simulink model "depth_lin"  (R2023b)
settings: Solver=VariableStepAuto  StartTime=0.0  StopTime=100  RelTol=1e-3
settings Model: Creator=fabio  LastModifiedBy=fabio

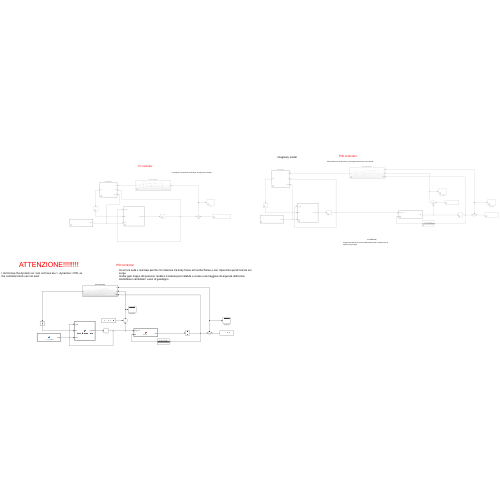
[thumbnail: Simulink's stored preview of the top-level diagram]
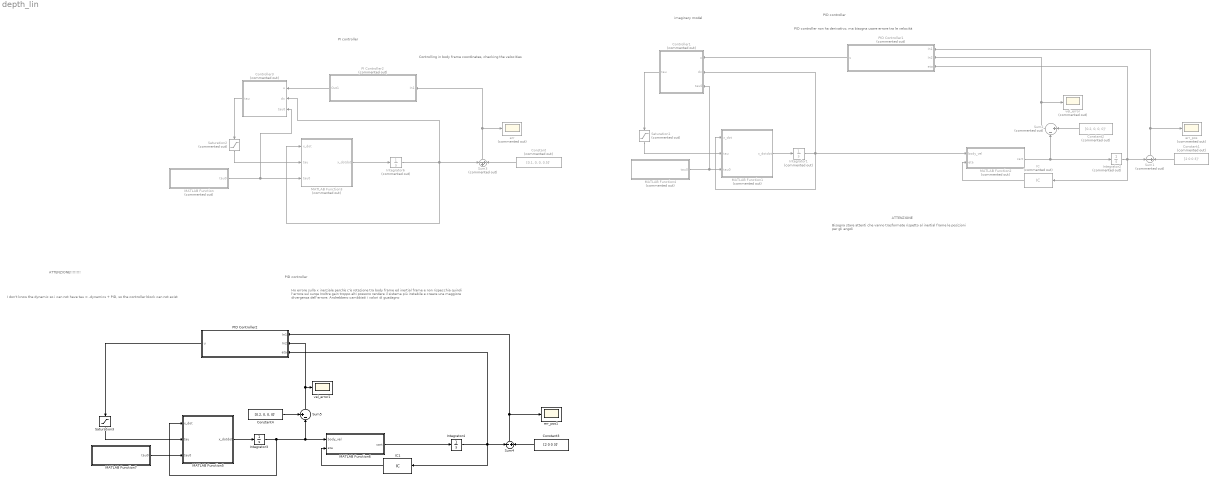
== system depth_lin ==
  note: Ho errore sulla x inerziale perchè c'è rotazione tra body frame ed inertial frame e non rispecchia quindi l'errore sul surge
      | Inoltre gain troppo alti possono rendere il sistema più instabile e creare una maggiore divergenza dell'errore.
      | Andrebbero cambbiati i valori di guadagno
  note: imaginary model
  note: I don't know the dynamic so i can not have tau = -dynamics + PID, so the controller block can not exist
  note: ATTENZIONE!!!!!!!!
  note: PID controller non ha derivativo, ma bisogna usare errore tra le velocità
  note: Controlling in body frame coordinates, checking the velocities
  note: PID controller
  note: PI controller
  note: Bisogna stare attenti che vanno trasformate rispetto al inertial frame le posizioni per gli angoli
  note: ATTENZIONE
  note: PID controller
  Constant : Constant  Commented=on  Value=[0.1, 0, 0, 0.5]'
  Constant1 : Constant  Commented=on  Value=[2 0 0 3]'
  Constant2 : Constant  Commented=on  Value=[0.2, 0, 0, 0]'
  Constant3 : Constant  Value=[2 0 0 3]'
  Constant4 : Constant  Value=[0.2, 0, 0, 0]'
  Controller1 : MATLAB Function  Commented=on  TreatAsAtomicUnit=on
  Controller3 : MATLAB Function  Commented=on  TreatAsAtomicUnit=on
  IC : InitialCondition  Commented=on  Value=[1, 0, 1, 0.5]'
  IC1 : InitialCondition  Value=[1, 0, 0, 0.5]'
  Integrator1 : Integrator  Commented=on
  Integrator2 : Integrator  Commented=on
  Integrator3 : Integrator
  Integrator4 : Integrator
  Integrator6 : Integrator  Commented=on
  MATLAB Function : MATLAB Function  Commented=on  TreatAsAtomicUnit=on
  MATLAB Function1 : MATLAB Function  Commented=on  TreatAsAtomicUnit=on
  MATLAB Function2 : MATLAB Function  Commented=on  TreatAsAtomicUnit=on
  MATLAB Function3 : MATLAB Function  Commented=on  TreatAsAtomicUnit=on
  MATLAB Function4 : MATLAB Function  Commented=on  TreatAsAtomicUnit=on
  MATLAB Function5 : MATLAB Function  TreatAsAtomicUnit=on
  MATLAB Function6 : MATLAB Function  TreatAsAtomicUnit=on
  MATLAB Function7 : MATLAB Function  TreatAsAtomicUnit=on
  PI Controller2 : Subsystem  Commented=on
  PID Controller1 : Subsystem  Commented=on
  PID Controller2 : Subsystem
  Saturation1 : Saturate  Commented=on  UpperLimit=20000  LowerLimit=-20000
  Saturation2 : Saturate  Commented=on  UpperLimit=20000  LowerLimit=-20000
  Saturation3 : Saturate  UpperLimit=20000  LowerLimit=-20000
  Sum1 : Sum  Commented=on  Inputs=-+
  Sum2 : Sum  Commented=on  Inputs=||+|-
  Sum3 : Sum  Commented=on  Inputs=-++
  Sum4 : Sum  Inputs=-+
  Sum5 : Sum  Inputs=+-|
  err : Scope  Commented=on
  err_pos : Scope  Commented=on
  err_pos1 : Scope
  vel_error : Scope  Commented=on
  vel_error1 : Scope
  wires:
  Controller3/1(tau) -> Saturation2/1
  Sum3/1 -> err/1, PI Controller2/1(In1)
  Saturation2/1 -> MATLAB Function3/2(tau)
  PI Controller2/1(Out1) -> Controller3/1(u)
  MATLAB Function3/1(x_dotdot) -> Integrator6/1
  Integrator6/1 -> Controller3/2(dx), MATLAB Function3/1(x_dot), Sum3/1
  MATLAB Function2/1(cart) -> Sum2/2, Integrator2/1
  Controller1/1(tau) -> Saturation1/1
  Integrator2/1 -> PID Controller1/3(eta), IC/1, Sum1/1
  Saturation1/1 -> MATLAB Function1/2(tau)
  Integrator1/1 -> MATLAB Function2/1(body_vel), MATLAB Function1/1(x_dot), Controller1/2(dx)
  MATLAB Function1/1(x_dotdot) -> Integrator1/1
  Sum1/1 -> PID Controller1/1(In1), err_pos/1
  MATLAB Function/1(tau0) -> MATLAB Function3/3(tau0), Controller3/3(tau0)
  Constant/1 -> Sum3/3
  MATLAB Function4/1(tau0) -> MATLAB Function1/3(tau0), Controller1/3(tau0)
  Constant1/1 -> Sum1/2
  Sum2/1 -> PID Controller1/2(In2), vel_error/1
  Constant2/1 -> Sum2/1
  PID Controller1/1(u) -> Controller1/1(u)
  IC/1 -> MATLAB Function2/2(eta)
  Constant4/1 -> Sum5/1
  Constant3/1 -> Sum4/2
  Saturation3/1 -> MATLAB Function5/2(tau)
  Integrator3/1 -> MATLAB Function6/1(body_vel), Sum5/2, MATLAB Function5/1(x_dot)
  Sum5/1 -> PID Controller2/2(In2), vel_error1/1
  MATLAB Function5/1(x_dotdot) -> Integrator3/1
  IC1/1 -> MATLAB Function6/2(eta)
  MATLAB Function7/1(tau0) -> MATLAB Function5/3(tau0)
  Integrator4/1 -> PID Controller2/3(eta), IC1/1, Sum4/1
  Sum4/1 -> PID Controller2/1(In1), err_pos1/1
  MATLAB Function6/1(cart) -> Integrator4/1
  PID Controller2/1(u) -> Saturation3/1

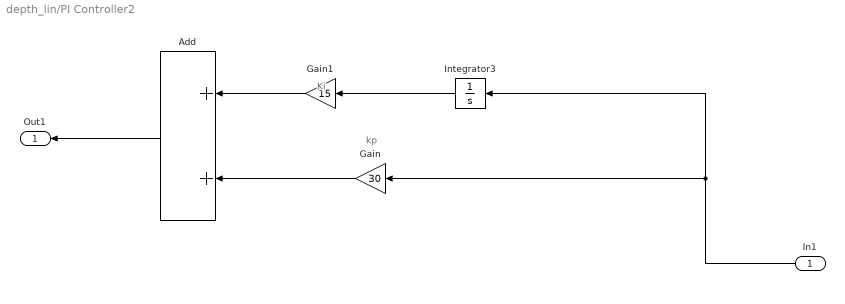
== system depth_lin/PI Controller2 ==
  note: Ki
  note: kp
  In1 : Inport
  Add : Sum
  Gain : Gain  Gain=30
  Gain1 : Gain  Gain=15
  Integrator3 : Integrator
  Out1 : Outport
  wires:
  Gain/1 -> Add/2
  Integrator3/1 -> Gain1/1
  In1/1 -> Integrator3/1, Gain/1
  Add/1 -> Out1/1
  Gain1/1 -> Add/1

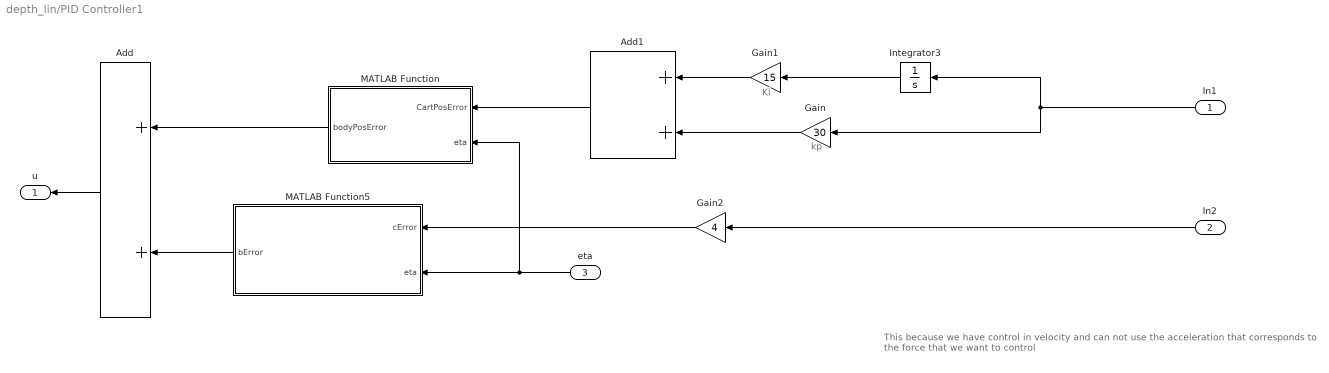
== system depth_lin/PID Controller1 ==
  note: This because we have control in velocity and can not use the acceleration that corresponds to the force that we want to control
  note: Ki
  note: kp
  In1 : Inport
  In2 : Inport  Port=2
  eta : Inport  Port=3
  Add : Sum
  Add1 : Sum
  Gain : Gain  Gain=30
  Gain1 : Gain  Gain=15
  Gain2 : Gain  Gain=4
  Integrator3 : Integrator
  MATLAB Function : MATLAB Function  TreatAsAtomicUnit=on
  MATLAB Function5 : MATLAB Function  TreatAsAtomicUnit=on
  u : Outport
  wires:
  Integrator3/1 -> Gain1/1
  In1/1 -> Integrator3/1, Gain/1
  Add/1 -> u/1
  In2/1 -> Gain2/1
  Gain1/1 -> Add1/1
  Gain/1 -> Add1/2
  Gain2/1 -> MATLAB Function5/1(cError)
  MATLAB Function5/1(bError) -> Add/2
  eta/1 -> MATLAB Function/2(eta), MATLAB Function5/2(eta)
  Add1/1 -> MATLAB Function/1(CartPosError)
  MATLAB Function/1(bodyPosError) -> Add/1

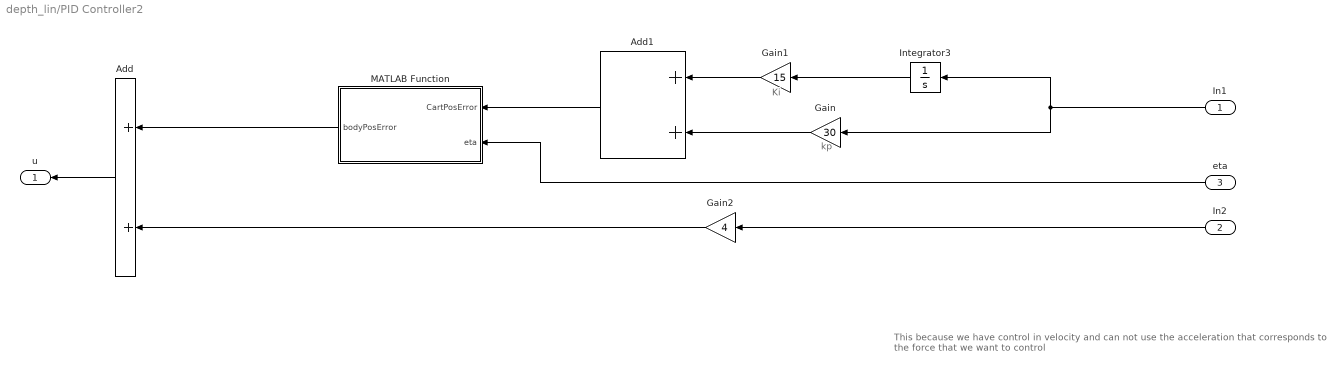
== system depth_lin/PID Controller2 ==
  note: This because we have control in velocity and can not use the acceleration that corresponds to the force that we want to control
  note: Ki
  note: kp
  In1 : Inport
  In2 : Inport  Port=2
  eta : Inport  Port=3
  Add : Sum
  Add1 : Sum
  Gain : Gain  Gain=30
  Gain1 : Gain  Gain=15
  Gain2 : Gain  Gain=4
  Integrator3 : Integrator
  MATLAB Function : MATLAB Function  TreatAsAtomicUnit=on
  u : Outport
  wires:
  Integrator3/1 -> Gain1/1
  In1/1 -> Integrator3/1, Gain/1
  Add/1 -> u/1
  In2/1 -> Gain2/1
  Gain1/1 -> Add1/1
  Gain/1 -> Add1/2
  Gain2/1 -> Add/2
  eta/1 -> MATLAB Function/2(eta)
  Add1/1 -> MATLAB Function/1(CartPosError)
  MATLAB Function/1(bodyPosError) -> Add/1

== matlab function depth_lin/MATLAB Function7 ==
  data: tau0 output
function tau0 = tau0Computation()
    % updated to medusa model
    m = 30;
    I = 4.14;
    g = 9.81;
    WB = -0.8339; % Buoyancy
    
    % x initial
    speed0 = [0.1, 0, 0, 0]';

    % Added mass
    tau_a = [-25; -2.325; -8.690; -19.4311]; % kl_dot

    % Restoring forces
    tau_r = [-0.2; -55.117; -4.14; 33.6804]; % kl

    % Hydrodynamic forces
    tau_d = [-19.5; -147.9; -6.23; -89.4105]; % kl_modl

    % Virtual mass
    mv = [m; m; I; m] - tau_a;

    % Dissatipative forces
    dv = -tau_r - 2*tau_d .* abs(speed0);
    
    % tau0 computation
    tau0 = zeros(4,1);
    tau0(1) = dv(1)*speed0(1) - mv(2)*speed0(2)*speed0(3);
    tau0(2) = 0; % can do also the equations
    tau0(3) = dv(3)*speed0(3) - (mv(1) - mv(2))*speed0(1)*speed0(2);
    tau0(4) = -dv(4)*speed0(4) - WB;
end

== matlab function depth_lin/PID Controller2/MATLAB Function ==
  data: CartPosError input; bodyPosError output; eta input
function bodyPosError = Rotation(CartPosError, eta)
    angle = eta(3);
    bodyPosError = zeros(4,1);
    rot = [cos(angle), -sin(angle)
            sin(angle), cos(angle)];

    bodyPosError(1:2) = rot' * CartPosError(1:2);
    bodyPosError(3:4) = CartPosError(3:4);
end

== matlab function depth_lin/Controller1 ==
  data: u input; dx input; tau output; tau0 input
function tau = controller(u, dx, tau0)
    % updated to medusa model
    m = 30;
    I = 4.14;
    K = 1;
    
    % x initial
    speed0 = [0.1, 0, 0, 0]';

    % Added mass
    tau_a = [-25; -2.325; -8.690; -19.4311]; % kl_dot

    % Restoring forces
    tau_r = [-0.2; -55.117; -4.14; 33.6804]; % kl

    % Hydrodynamic forces
    tau_d = [-19.5; -147.9; -6.23; -89.4105]; % kl_modl

    % Virtual mass
    mv = [m; m; I; m] - tau_a;

    % Dissatipative forces
    dv = -tau_r - 2*tau_d .*abs(speed0);
    
    % delta velocities
    delta = dx - speed0;
    % Accelerations
    % 3 DOF MODEL
    tau = zeros(4,1);
    % Tested tau. Which is the best methods??
    % tau(1) = mv(1)*K*u(1) + dv(1)*dx(1) - mv(2)*speed0(2)*dx(3) - mv(2)*speed0(3)*dx(2);
    % tau(2) = 0; % can do also the equations
    % tau(3) = mv(3)*K*u(3) + dv(3)*dx(3) - (mv(1) - mv(2))*speed0(1)*dx(2) - (mv(1) - mv(2))*speed0(2)*dx(1);
    % % Considering also depth (heavy)
    % tau(4) =  mv(4)*K*u(4) - dv(4)*dx(4);

    % Consider also deltas and initial tau
    tau(1) = mv(1)*K*u(1) + dv(1)*delta(1) - mv(2)*speed0(2)*delta(3) - mv(2)*speed0(3)*delta(2) + tau0(1);
    tau(2) = 0; % can do also the equations
    tau(3) = mv(3)*K*u(3) + dv(3)*delta(3) - (mv(1) - mv(2))*speed0(1)*delta(2) - (mv(1) - mv(2))*speed0(2)*delta(1) + tau0(3);
    % Considering also depth (heavy)
    tau(4) =  mv(4)*K*u(4) - dv(4)*delta(4) + tau0(4);
end

== matlab function depth_lin/MATLAB Function1 ==
  data: x_dot input; tau input; tau0 input; x_dotdot output
function x_dotdot = vehicle_dynamics_matrix(x_dot, tau, tau0)
    % updated to medusa model
    m = 30;
    I = 4.14;
    
    % x initial
    speed0 = [0.1, 0, 0, 0]';

    % Added mass
    tau_a = [-25; -2.325; -8.690; -19.4311]; % kl_dot

    % Restoring forces
    tau_r = [-0.2; -55.117; -4.14; 33.6804]; % kl

    % Hydrodynamic forces
    tau_d = [-19.5; -147.9; -6.23; -89.4105]; % kl_modl

    % Virtual mass
    mv = [m; m; I; m] - tau_a;

    % Dissatipative forces
    dv = -tau_r - 2*tau_d .* abs(speed0);

    delta = x_dot - speed0;

    % Accelerations
    % 3 DOF MODEL Linearized
    x_dotdot = zeros(4,1);
    x_dotdot(1) = (tau(1) - tau0(1) - dv(1)*delta(1) + mv(2)*speed0(2)*delta(3) + mv(2)*speed0(3)*delta(2)) / mv(1); 
    x_dotdot(2) = (tau(2) - tau0(2) - dv(2)*delta(2) - mv(1)*speed0(1)*delta(3) - mv(1)*speed0(3)*delta(1)) / mv(2);
    x_dotdot(3) = (tau(3) - tau0(3) - dv(3)*delta(3) + (mv(1) - mv(2))*speed0(1)*delta(2) + (mv(1) - mv(2))*speed0(2)*delta(1)) / mv(3);
    % Considering also depth (heavy)
    x_dotdot(4) = (tau(4) - tau0(4) + dv(4)*delta(4)) / mv(4);
end

== matlab function depth_lin/MATLAB Function2 ==
  data: cart output; body_vel input; eta input
function cart = mapping(body_vel, eta)
    cart = zeros(4,1);
    Jacobian = eye(4);
    angle = eta(3);
    Jacobian(1:2, 1:2) = [cos(angle), -sin(angle);
                          sin(angle), cos(angle)];
    cart = Jacobian * body_vel;
end

== matlab function depth_lin/MATLAB Function ==
  data: tau0 output
function tau0 = tau0Computation()
    % updated to medusa model
    m = 30;
    I = 4.14;
    g = 9.81;
    WB = -0.8339; % Buoyancy
    
    % x initial
    speed0 = [0.1, 0, 0, 0]';

    % Added mass
    tau_a = [-25; -2.325; -8.690; -19.4311]; % kl_dot

    % Restoring forces
    tau_r = [-0.2; -55.117; -4.14; 33.6804]; % kl

    % Hydrodynamic forces
    tau_d = [-19.5; -147.9; -6.23; -89.4105]; % kl_modl

    % Virtual mass
    mv = [m; m; I; m] - tau_a;

    % Dissatipative forces
    dv = -tau_r - 2*tau_d .* abs(speed0);
    
    % tau0 computation
    tau0 = zeros(4,1);
    tau0(1) = dv(1)*speed0(1) - mv(2)*speed0(2)*speed0(3);
    tau0(2) = 0; % can do also the equations
    tau0(3) = dv(3)*speed0(3) - (mv(1) - mv(2))*speed0(1)*speed0(2);
    tau0(4) = -dv(4)*speed0(4) - WB;
end

== matlab function depth_lin/MATLAB Function4 ==
  data: tau0 output
function tau0 = tau0Computation()
    % updated to medusa model
    m = 30;
    I = 4.14;
    g = 9.81;
    WB = -0.8339; % Buoyancy
    
    % x initial
    speed0 = [0.1, 0, 0, 0]';

    % Added mass
    tau_a = [-25; -2.325; -8.690; -19.4311]; % kl_dot

    % Restoring forces
    tau_r = [-0.2; -55.117; -4.14; 33.6804]; % kl

    % Hydrodynamic forces
    tau_d = [-19.5; -147.9; -6.23; -89.4105]; % kl_modl

    % Virtual mass
    mv = [m; m; I; m] - tau_a;

    % Dissatipative forces
    dv = -tau_r - 2*tau_d .* abs(speed0);
    
    % tau0 computation
    tau0 = zeros(4,1);
    tau0(1) = dv(1)*speed0(1) - mv(2)*speed0(2)*speed0(3);
    tau0(2) = 0; % can do also the equations
    tau0(3) = dv(3)*speed0(3) - (mv(1) - mv(2))*speed0(1)*speed0(2);
    tau0(4) = -dv(4)*speed0(4) - WB;
end

== matlab function depth_lin/PID Controller1/MATLAB Function5 ==
  data: cError input; bError output; eta input
function bError = InverseMapping(cError, eta)
    % Jacobian = eye(4);
    bError = zeros(4,1);
    angle = eta(3);
    Jacobian = [cos(angle), -sin(angle);
                  sin(angle), cos(angle)];
    bError(1:2) = pinv(Jacobian) * cError(1:2);
    bError(3:4) = cError(3:4);
end

== matlab function depth_lin/PID Controller1/MATLAB Function ==
  data: CartPosError input; bodyPosError output; eta input
function bodyPosError = Rotation(CartPosError, eta)
    angle = eta(3);
    bodyPosError = zeros(4,1);
    rot = [cos(angle), -sin(angle)
            sin(angle), cos(angle)];

    bodyPosError(1:2) = rot' * CartPosError(1:2);
    bodyPosError(3:4) = CartPosError(3:4);
end

== matlab function depth_lin/MATLAB Function5 ==
  data: x_dot input; tau input; tau0 input; x_dotdot output
function x_dotdot = vehicle_dynamics_matrix(x_dot, tau, tau0)
    % updated to medusa model
    m = 30;
    I = 4.14;
    
    % x initial
    speed0 = [0.1, 0, 0, 0]';

    % Added mass
    tau_a = [-25; -2.325; -8.690; -19.4311]; % kl_dot

    % Restoring forces
    tau_r = [-0.2; -55.117; -4.14; 33.6804]; % kl

    % Hydrodynamic forces
    tau_d = [-19.5; -147.9; -6.23; -89.4105]; % kl_modl

    % Virtual mass
    mv = [m; m; I; m] - tau_a;

    % Dissatipative forces
    dv = -tau_r - 2*tau_d .* abs(speed0);

    delta = x_dot - speed0;

    % Accelerations
    % 3 DOF MODEL Linearized
    x_dotdot = zeros(4,1);
    x_dotdot(1) = (tau(1) - tau0(1) - dv(1)*delta(1) + mv(2)*speed0(2)*delta(3) + mv(2)*speed0(3)*delta(2)) / mv(1); 
    x_dotdot(2) = (tau(2) - tau0(2) - dv(2)*delta(2) - mv(1)*speed0(1)*delta(3) - mv(1)*speed0(3)*delta(1)) / mv(2);
    x_dotdot(3) = (tau(3) - tau0(3) - dv(3)*delta(3) + (mv(1) - mv(2))*speed0(1)*delta(2) + (mv(1) - mv(2))*speed0(2)*delta(1)) / mv(3);
    % Considering also depth (heavy)
    x_dotdot(4) = (tau(4) - tau0(4) + dv(4)*delta(4)) / mv(4);
end

== matlab function depth_lin/Controller3 ==
  data: u input; dx input; tau output; tau0 input
function tau = controller(u, dx, tau0)
    % updated to medusa model
    m = 30;
    I = 4.14;
    K = 1;
    
    % x initial
    speed0 = [0.1, 0, 0, 0]';

    % Added mass
    tau_a = [-25; -2.325; -8.690; -19.4311]; % kl_dot

    % Restoring forces
    tau_r = [-0.2; -55.117; -4.14; 33.6804]; % kl

    % Hydrodynamic forces
    tau_d = [-19.5; -147.9; -6.23; -89.4105]; % kl_modl

    % Virtual mass
    mv = [m; m; I; m] - tau_a;

    % Dissatipative forces
    dv = -tau_r - 2*tau_d .*abs(speed0);
    
    % delta velocities
    delta = dx - speed0;
    % Accelerations
    %% 3 DOF MODEL
    tau = zeros(4,1);
    % Tested tau. Which is the best methods??
    % tau(1) = mv(1)*K*u(1) + dv(1)*dx(1) - mv(2)*speed0(2)*dx(3) - mv(2)*speed0(3)*dx(2);
    % tau(2) = 0; % can do also the equations
    % tau(3) = mv(3)*K*u(3) + dv(3)*dx(3) - (mv(1) - mv(2))*speed0(1)*dx(2) - (mv(1) - mv(2))*speed0(2)*dx(1);
    % % Considering also depth (heavy)
    % tau(4) =  mv(4)*K*u(4) - dv(4)*dx(4);

    % Consider also deltas and initial tau
    tau(1) = mv(1)*K*u(1) + dv(1)*delta(1) - mv(2)*speed0(2)*delta(3) - mv(2)*speed0(3)*delta(2) + tau0(1);
    tau(2) = 0; % can do also the equations
    tau(3) = mv(3)*K*u(3) + dv(3)*delta(3) - (mv(1) - mv(2))*speed0(1)*delta(2) - (mv(1) - mv(2))*speed0(2)*delta(1) + tau0(3);
    % Considering also depth (heavy)
    tau(4) =  mv(4)*K*u(4) - dv(4)*delta(4) + tau0(4);
end

== matlab function depth_lin/MATLAB Function3 ==
  data: x_dot input; tau input; x_dotdot output; tau0 input
function x_dotdot = vehicle_dynamics_matrix(x_dot, tau, tau0)
    % updated to medusa model
    m = 30;
    I = 4.14;
    
    % x initial
    speed0 = [0.1, 0, 0, 0]';

    % Added mass
    tau_a = [-25; -2.325; -8.690; -19.4311]; % kl_dot

    % Restoring forces
    tau_r = [-0.2; -55.117; -4.14; 33.6804]; % kl

    % Hydrodynamic forces
    tau_d = [-19.5; -147.9; -6.23; -89.4105]; % kl_modl

    % Virtual mass
    mv = [m; m; I; m] - tau_a;

    % Dissatipative forces
    dv = -tau_r - 2*tau_d .* abs(speed0);

    delta = x_dot - speed0;

    % Accelerations
    % 3 DOF MODEL Linearized
    x_dotdot = zeros(4,1);
    x_dotdot(1) = (tau(1) - tau0(1) - dv(1)*delta(1) + mv(2)*speed0(2)*delta(3) + mv(2)*speed0(3)*delta(2)) / mv(1); 
    x_dotdot(2) = (tau(2) - tau0(2) - dv(2)*delta(2) - mv(1)*speed0(1)*delta(3) - mv(1)*speed0(3)*delta(1)) / mv(2);
    x_dotdot(3) = (tau(3) - tau0(3) - dv(3)*delta(3) + (mv(1) - mv(2))*speed0(1)*delta(2) + (mv(1) - mv(2))*speed0(2)*delta(1)) / mv(3);
    % Considering also depth (heavy)
    x_dotdot(4) = (tau(4) - tau0(4) + dv(4)*delta(4)) / mv(4);

== matlab function depth_lin/MATLAB Function6 ==
  data: cart output; body_vel input; eta input
function cart = mapping(body_vel, eta)
    Jacobian = eye(4);
    angle = eta(3);
    Jacobian(1:2, 1:2) = [cos(angle), -sin(angle);
                          sin(angle), cos(angle)];
    cart = Jacobian * body_vel;
end
